simulink model "sistema_mecanico"  (R2018a)
settings: Solver=VariableStepAuto  StartTime=0.0  StopTime=10.0  RelTol=1e-3
values from neighbouring files (symbols this model uses):
  B1 = 40    [ejemplo_mecanico.m]    (also in veengranes.m = 10)
  B2 = 20    [ejemplo_mecanico.m]    (also in veengranes.m = 34)
  B3 = 10    [ejemplo_mecanico.m]
  k1 = 100    [anexo_parcial.m]    (also in ejemplo_mecanico.m)
  k2 = 300    [anexo_parcial.m]    (also in ejemplo_mecanico.m = 400)
  k3 = 150    [ejemplo_mecanico.m]
  M1 = 10    [ejemplo_mecanico.m]
  M2 = 30    [ejemplo_mecanico.m]
settings Model: Creator=carma  LastModifiedBy=carma

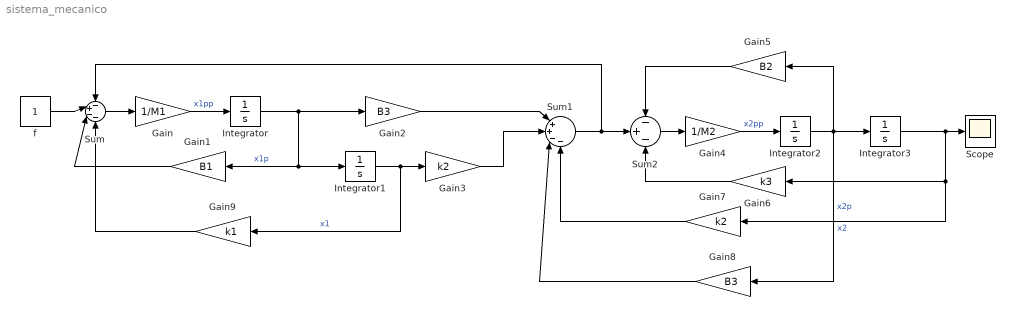
== system sistema_mecanico ==
  Gain : Gain  Gain=1/M1
  Gain1 : Gain  Gain=B1
  Gain2 : Gain  Gain=B3
  Gain3 : Gain  Gain=k2
  Gain4 : Gain  Gain=1/M2
  Gain5 : Gain  Gain=B2
  Gain6 : Gain  Gain=k3
  Gain7 : Gain  Gain=k2
  Gain8 : Gain  Gain=B3
  Gain9 : Gain  Gain=k1
  Integrator{,1..3} (4 alike) : Integrator
  Scope : Scope
  Sum : Sum  Inputs=-+--
  Sum1 : Sum  Inputs=|++--
  Sum2 : Sum  Inputs=-+-
  f : Constant
  wires:
  Sum/1 -> Gain/1
  Gain1/1 -> Sum/3
  Gain/1 -> Integrator/1  "x1pp"
  Integrator/1 -> Integrator1/1, Gain1/1, Gain2/1  "x1p"
  Gain2/1 -> Sum1/1
  Integrator1/1 -> Gain9/1, Gain3/1  "x1"
  Gain3/1 -> Sum1/2
  Sum1/1 -> Sum/1, Sum2/2
  Gain8/1 -> Sum1/3
  Gain7/1 -> Sum1/4
  f/1 -> Sum/2
  Gain4/1 -> Integrator2/1  "x2pp"
  Sum2/1 -> Gain4/1
  Integrator2/1 -> Gain8/1, Gain5/1, Integrator3/1  "x2p"
  Integrator3/1 -> Gain7/1, Gain6/1, Scope/1  "x2"
  Gain5/1 -> Sum2/1
  Gain6/1 -> Sum2/3
  Gain9/1 -> Sum/4
